simulink model "UnicycleWithSensor"  (R2025b)
settings: Solver=VariableStepAuto  StartTime=0.0  StopTime=200  RelTol=1e-3
values from neighbouring files (symbols this model uses):
  l = 0.5    [go2goalWithSensor.m]
  P = 10    [go2goalWithSensor.m]
  r = 0.1    [go2goalWithSensor.m]
  thetainit = 0    [go2goalWithSensor.m]
  tol = 0.1    [go2goalWithSensor.m]
  v = 0.5    [go2goalWithSensor.m]
  xg = gPos(2)    [go2goalWithSensor.m]
  xinit = sPos(2)    [go2goalWithSensor.m]
  yg = gPos(1)    [go2goalWithSensor.m]
  yinit = sPos(1)    [go2goalWithSensor.m]
  Z = ones(SizeX, SizeY)*255    [CreateMaze.m]
libraries: slpidlib x1, simulink_extras x1
settings Model: PacingRate=4  Creator=npn01  LastModifiedBy=kimsv
settings SolverCC: AlgebraicLoopSolver=TrustRegion
settings DebuggingCC: UnconnectedInputMsg=warning  UnconnectedOutputMsg=warning  UnconnectedLineMsg=warning  ArithmeticOperatorsInVariantConditions=warning
settings ModelReferenceCC: EnableRefExpFcnMdlSchedulingChecks=on
settings SFSimCC: CustomCodeUndefinedFunction=UseInterfaceOnly
settings RTWCC: GPUComputeCapability=3.5

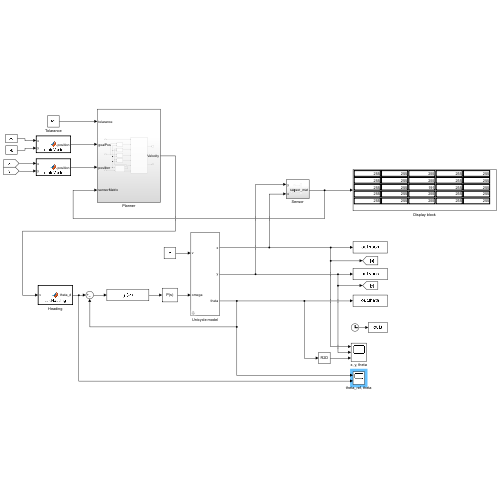
[thumbnail: Simulink's stored preview of the top-level diagram]
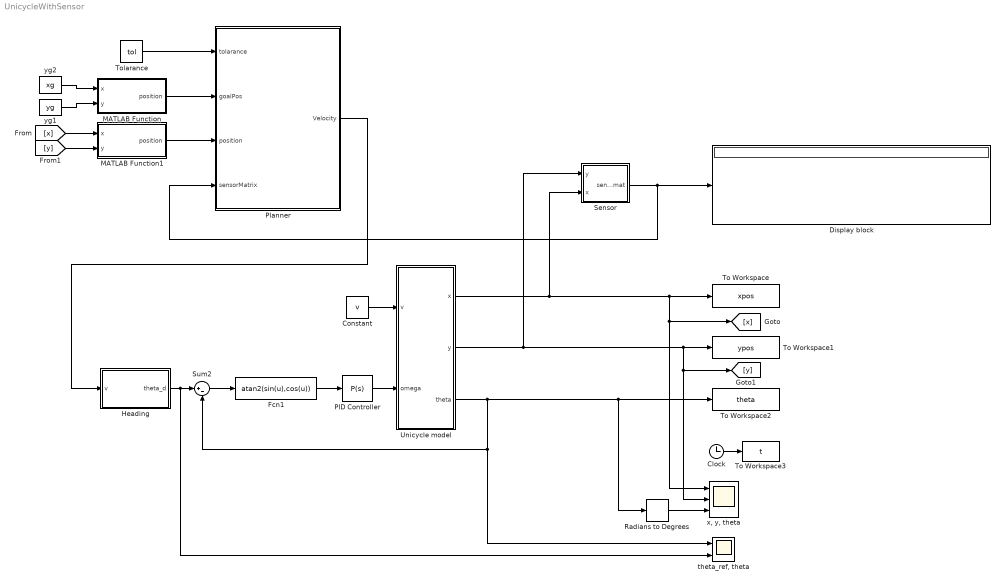
== system UnicycleWithSensor ==
  Clock : Clock
  Constant : Constant  Value=v
  Display block : Display
  Fcn1 : Fcn  Expr=atan2(sin(u),cos(u))
  Heading : MATLAB Function  TreatAsAtomicUnit=on
  MATLAB Function : MATLAB Function  TreatAsAtomicUnit=on
  MATLAB Function1 : MATLAB Function  TreatAsAtomicUnit=on
  PID Controller : slpidlib/PID Controller  Controller=P  Form=Parallel  TimeDomain=Continuous-time  UseExternalTs=off  SampleTime=-1  IntegratorMethod=Forward Euler  FilterMethod=Forward Euler  ControllerParametersSource=internal  P=P  I=0  UseKiTs=off  D=0  UseExternalDerivativeSource=off  N=100  UseFilter=on  TunerSelectOption=Transfer Function Based (PID Tuner App)  InitialConditionSource=internal  InitialConditionForIntegrator=0  InitialConditionForFilter=0  DifferentiatorICPrevScaledInput=0  ExternalReset=none  TrackingMode=off  Kt=1  LimitOutput=off  SatLimitsSource=internal  UpperSaturationLimit=inf  LowerSaturationLimit=-inf  LinearizeAsGain=on  AntiWindupMode=none  Kb=1  LimitIntegrator=off  UpperIntegratorSaturationLimit=inf  LowerIntegratorSaturationLimit=-inf  POutMin=[]  POutMax=[]  IOutMin=[]  IOutMax=[]  DOutMin=[]  DOutMax=[]  NOutMin=[]  NOutMax=[]  SumOutMin=[]  SumOutMax=[]  SaturationOutMin=[]  SaturationOutMax=[]  PParamMin=[]  PParamMax=[]  IParamMin=[]  IParamMax=[]  DParamMin=[]  DParamMax=[]  NParamMin=[]  NParamMax=[]  KbParamMin=[]  KbParamMax=[]  KtParamMin=[]  KtParamMax=[]  KbOutMin=[]  KbOutMax=[]  KtOutMin=[]  KtOutMax=[]  IntegratorOutMin=[]  IntegratorOutMax=[]  FilterOutMin=[]  FilterOutMax=[]  SumI1OutMin=[]  SumI1OutMax=[]  SumI2OutMin=[]  SumI2OutMax=[]  SumI3OutMin=[]  SumI3OutMax=[]  SumI4OutMin=[]  SumI4OutMax=[]  SumDOutMin=[]  SumDOutMax=[]  DifferentiatorOutMin=[]  DifferentiatorOutMax=[]  FilterDiffOutCoefMin=[]  FilterDiffOutCoefMax=[]  ReciprocalOutMin=[]  ReciprocalOutMax=[]  SumDenOutMin=[]  SumDenOutMax=[]  SumNumOutMin=[]  SumNumOutMax=[]  DivideOutMin=[]  DivideOutMax=[]  UdiffTsProdOutMin=[]  UdiffTsProdOutMax=[]  NTsProdOutMin=[]  NTsProdOutMax=[]  UintegralTsProdOutMin=[]  UintegralTsProdOutMax=[]  UngainTsProdOutMin=[]  UngainTsProdOutMax=[]  ClampingZeroOutDataTypeStr=Inherit: Inherit via back propagation  ClampingZeroOutMin=[]  ClampingZeroOutMax=[]  FilterDenConstantOutDataTypeStr=Inherit: Inherit via back propagation  FilterDenConstantOutMin=[]  FilterDenConstantOutMax=[]  PCopyOutDataTypeStr=Inherit: Inherit via back propagation  PCopyOutMin=[]  PCopyOutMax=[]  NCopyOutDataTypeStr=Inherit: Inherit via back propagation  NCopyOutMin=[]  NCopyOutMax=[]  IntegratorContinuousStateAttributes=''  IntegratorStateMustResolveToSignalObject=off  IntegratorRTWStateStorageClass=Auto  FilterContinuousStateAttributes=''  FilterStateMustResolveToSignalObject=off  FilterRTWStateStorageClass=Auto  ParallelPVariant=InternalParameters  IdealPVariant=Disabled  IVariant=Disabled  DVariant=Disabled  IntegratorVariant=Disabled  SatVariant=Disabled  AWVariant=Disabled  PCopyVariant=Disabled  TRVariant=Disabled  FdbkBlocksVariant=Forward  IdealPFdbkVariant=Disabled  SatFdbkVariant=Disabled  DerivativeFilterVariant=Disabled  NVariant=Disabled  NCopyVariant=Disabled_SignalSpec  FilterICVariant=Disabled  IntegratorICVariant=Disabled  ExternalResetVariant=Disabled  TRSumVariant=Passthrough  SumFdbkVariant=Disabled  SumVariant=Passthrough_P  TsampFilterVariant=InternalTs  TsampNgainVariant=Passthrough  TsampIntegralVariant=Disabled_SignalSpec  ExternalSaturationOutDataTypeStr=Inherit: Same as second input  DerivativeSourceVariant=Disabled  PreIntVariant=InternalPreInt
  Planner : Subsystem
  Radians to Degrees : simulink_extras/Transformations/Radians to Degrees
  Sensor : Subsystem
  Sum2 : Sum  Inputs=|+-
  To Workspace : ToWorkspace  VariableName=xpos  SampleTime=-1
  To Workspace1 : ToWorkspace  VariableName=ypos  SampleTime=-1
  To Workspace2 : ToWorkspace  VariableName=theta  SampleTime=-1
  To Workspace3 : ToWorkspace  VariableName=t  SampleTime=-1
      settings: Save2DSignal=2-D array (concatenate along first dimension)
  Tolarance : Constant  Value=tol
  Unicycle model : Subsystem  mask{x0=xinit, y0=yinit, theta0=thetainit}
      mask DialogControl Control4 Prompt: Enter x initial position
      mask DialogControl Control2 Prompt: Enter y initial position
      mask DialogControl Control3 Prompt: Enter initial theta angle
      mask DialogControl Control6 Prompt: Any text you want
  "theta_ref, theta" : Scope  NumInputPorts=2
      settings: ActiveDisplayYMinimum=-3.6016873206532476  ActiveDisplayYMaximum=5.63573543998936
  "x, y, theta" : Scope  NumInputPorts=3
      settings: ActiveDisplayString=3  ActiveDisplayYMinimum=-134.97289881582088  ActiveDisplayYMaximum=314.97179029887303  YLabel=Angle (Degrees)  DataLoggingVariableName=ScopeData2
  yg1 : Constant  Value=yg
  yg2 : Constant  Value=xg
  wires:
  Unicycle model/1(x) -> Sensor/2(x), [x], "x, y, theta"/1, To Workspace/1
  Unicycle model/2(y) -> [y], "x, y, theta"/2, To Workspace1/1, Sensor/1(y)
  Unicycle model/3(theta) -> Radians to Degrees/1, To Workspace2/1, Sum2/2, "theta_ref, theta"/1
  PID Controller/1 -> Unicycle model/2(omega)
  Clock/1 -> To Workspace3/1
  Sensor/1(sensor_mat) -> Planner/4(sensorMatrix), Display block/1
  yg1/1 -> MATLAB Function/2(y)
  MATLAB Function/1(position) -> Planner/2(goalPos)
  MATLAB Function1/1(position) -> Planner/3(position)
  Planner/1(Velocity) -> Heading/1(v)
  Heading/1(theta_d) -> "theta_ref, theta"/2, Sum2/1
  [x] -> MATLAB Function1/1(x)
  [y] -> MATLAB Function1/2(y)
  Sum2/1 -> Fcn1/1
  Fcn1/1 -> PID Controller/1
  yg2/1 -> MATLAB Function/1(x)
  Radians to Degrees/1 -> "x, y, theta"/3
  Constant/1 -> Unicycle model/1(v)
  Tolarance/1 -> Planner/1(tolarance)

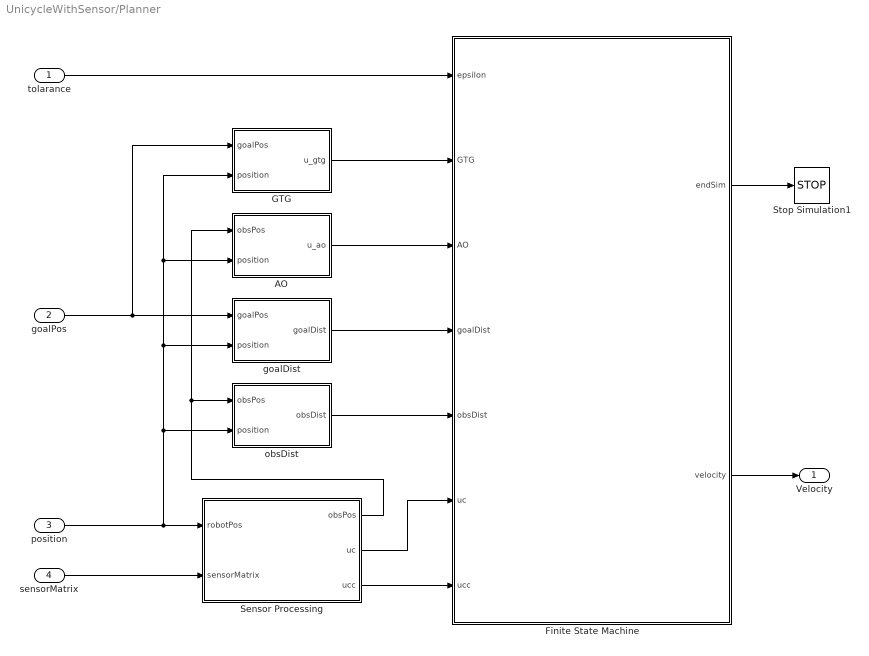
== system UnicycleWithSensor/Planner ==
  tolarance : Inport
  goalPos : Inport  Port=2
  position : Inport  Port=3
  sensorMatrix : Inport  Port=4
  AO : MATLAB Function  TreatAsAtomicUnit=on
  Finite State Machine : Stateflow chart  TreatAsAtomicUnit=on
      settings: PortSchema="{\"entries\":[{\"content\":{\"sides\":[{\"content\":{\"connectorIds\":[\"In7\",\"In3\",\"In4\",\"In5\",\"In6\",\"In1\",\"In2\"]},\"type\":\"ConnectorPlacement.EquallySpacedRectSide\",\"uuid\":\"7bddc3d5-5a53-4f00-97fb-67b91d40fd27\"},{\"content\":{\"connectorIds\":[\"Out2\",\"Out1\"],\"side\":\"RIGHT\"},\"type\":\"ConnectorPlacement.EquallySpacedRectSide\",\"uuid\":\"08b6080d-a441-42a3-994a-8d28211d42e3\"},{\"content\":{\"side\":\"TOP\"},\"type\":\"ConnectorPlacement.EquallySpacedRectSide\",\"uuid\":\"62170fc2-3338-4bec-a116-8b710f92c3e1\"}]},\"type\":\"ConnectorPlacement.EquallySpacedConnector\",\"uuid\":\"879b9b83-d19d-42da-995b-71e8b8a5ae61\"}],\"packageUris\":[\"http://schema.mathworks.com/mf0/Connector/R2020b\"],\"version\":\"1.0\"}"
  GTG : MATLAB Function  TreatAsAtomicUnit=on
  Sensor Processing : MATLAB Function  TreatAsAtomicUnit=on
  Stop Simulation1 : Stop
  goalDist : MATLAB Function  TreatAsAtomicUnit=on
  obsDist : MATLAB Function  TreatAsAtomicUnit=on
  Velocity : Outport
  wires:
  position/1 -> Sensor Processing/1(robotPos), obsDist/2(position), goalDist/2(position), AO/2(position), GTG/2(position)
  goalPos/1 -> GTG/1(goalPos), goalDist/1(goalPos)
  Sensor Processing/2(uc) -> Finite State Machine/1(uc)
  Sensor Processing/3(ucc) -> Finite State Machine/2(ucc)
  sensorMatrix/1 -> Sensor Processing/2(sensorMatrix)
  Sensor Processing/1(obsPos) -> AO/1(obsPos), obsDist/1(obsPos)
  GTG/1(u_gtg) -> Finite State Machine/3(GTG)
  goalDist/1(goalDist) -> Finite State Machine/5(goalDist)
  obsDist/1(obsDist) -> Finite State Machine/6(obsDist)
  Finite State Machine/2(endSim) -> Stop Simulation1/1
  Finite State Machine/1(velocity) -> Velocity/1
  tolarance/1 -> Finite State Machine/7(epsilon)
  AO/1(u_ao) -> Finite State Machine/4(AO)

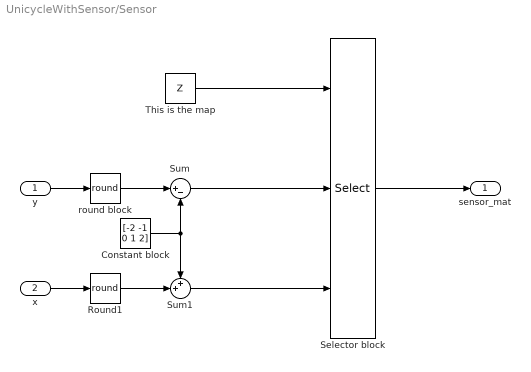
== system UnicycleWithSensor/Sensor ==
  y : Inport
  x : Inport  Port=2
  Constant block : Constant  Value=[-2 -1 0 1 2]
  Round1 : Rounding  Operator=round
  Selector block : Selector  NumberOfDimensions=2  InputPortWidth=3  IndexOptions=Index vector (port),Index vector (port)  Indices=[1 3],1  OutputSizes=1,1
  Sum : Sum  Inputs=|+-  OutDataTypeStr=int32  RndMeth=Round
  Sum1 : Sum  Inputs=++|  OutDataTypeStr=int32  RndMeth=Round
  This is the map : Constant  Value=Z  VectorParams1D=off
  round block : Rounding  Operator=round
  sensor_mat : Outport
  wires:
  This is the map/1 -> Selector block/1
  Constant block/1 -> Sum1/1, Sum/2
  Sum/1 -> Selector block/2
  Sum1/1 -> Selector block/3
  Selector block/1 -> sensor_mat/1
  y/1 -> round block/1
  round block/1 -> Sum/1
  x/1 -> Round1/1
  Round1/1 -> Sum1/2

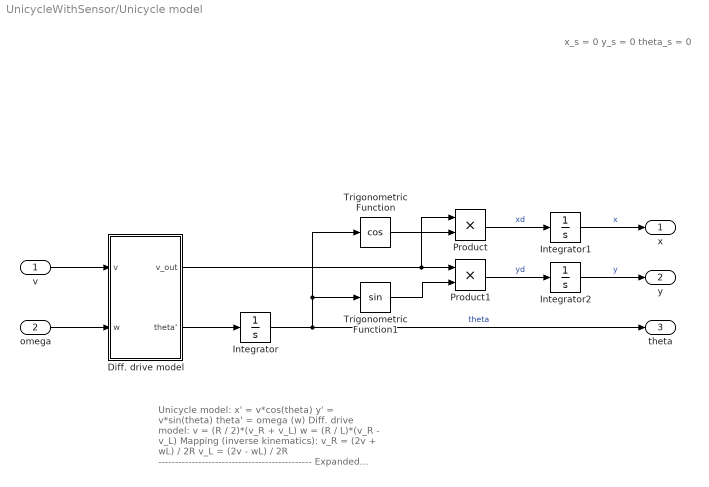
== system UnicycleWithSensor/Unicycle model ==
  note: x_s = 0
      | y_s = 0
      | theta_s = 0
  note: Unicycle model:
      | x' = v*cos(theta)
      | y' = v*sin(theta)
      | theta' = omega (w)
      |
      | Diff. drive model:
      | v = (R / 2)*(v_R + v_L)
      | w = (R / L)*(v_R - v_L)
      |
      | Mapping (inverse kinematics):
      | v_R = (2v + wL) / 2R
      | v_L = (2v - wL) / 2R
      | ----------------------------------------------
      | Expanded unicycle model:
      | x' =  ((R / 2)*(v_R + v_L))*cos(theta)
      | y' =  ((R / 2)*(v_R + v_L))*sin(theta)
      | theta' =  (R / L)*(v_R - v_L)
  v : Inport
  omega : Inport  Port=2
  Diff. drive model : Subsystem
  Integrator : Integrator  InitialCondition=theta0
  Integrator1 : Integrator  InitialCondition=x0
  Integrator2 : Integrator  InitialCondition=y0
  Product : Product
  Product1 : Product
  Trigonometric Function : Trigonometry  Operator=cos
  Trigonometric Function1 : Trigonometry
  x : Outport
  y : Outport  Port=2
  theta : Outport  Port=3
  wires:
  Product1/1 -> Integrator2/1  "yd"
  Integrator2/1 -> y/1  "y"
  v/1 -> Diff. drive model/1(v)
  Integrator/1 -> Trigonometric Function/1, Trigonometric Function1/1, theta/1  "theta"
  Product/1 -> Integrator1/1  "xd"
  omega/1 -> Diff. drive model/2(w)
  Trigonometric Function/1 -> Product/2
  Integrator1/1 -> x/1  "x"
  Trigonometric Function1/1 -> Product1/2
  Diff. drive model/1(v_out) -> Product/1, Product1/1
  Diff. drive model/2(theta') -> Integrator/1

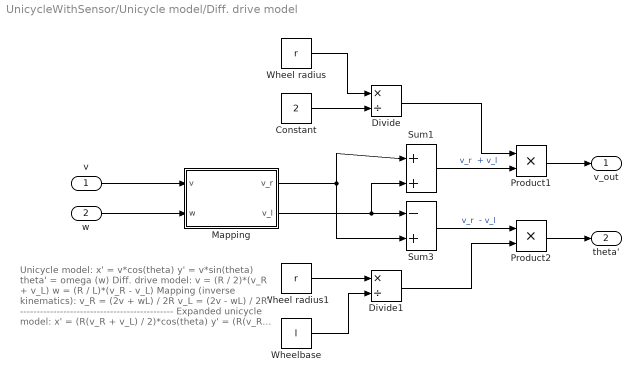
== system UnicycleWithSensor/Unicycle model/Diff. drive model ==
  note: Unicycle model:
      | x' = v*cos(theta)
      | y' = v*sin(theta)
      | theta' = omega (w)
      |
      | Diff. drive model:
      | v = (R / 2)*(v_R + v_L)
      | w = (R / L)*(v_R - v_L)
      |
      | Mapping (inverse kinematics):
      | v_R = (2v + wL) / 2R
      | v_L = (2v - wL) / 2R
      | ----------------------------------------------
      | Expanded unicycle model:
      | x' =  (R(v_R + v_L) / 2)*cos(theta)
      | y' =  (R(v_R + v_L) / 2)*sin(theta)
      | theta' =  R(v_R - v_L) / L
  v : Inport
  w : Inport  Port=2
  Constant : Constant  Value=2
  Divide : Product  Inputs=*/
  Divide1 : Product  Inputs=*/
  Mapping : Subsystem
  Product1 : Product
  Product2 : Product
  Sum1 : Sum  Inputs=+|+
  Sum3 : Sum  Inputs=-+
  Wheel radius : Constant  Value=r
  Wheel radius1 : Constant  Value=r
  Wheelbase : Constant  Value=l
  v_out : Outport
  theta' : Outport  Port=2
  wires:
  v/1 -> Mapping/1(v)
  w/1 -> Mapping/2(w)
  Wheel radius/1 -> Divide/1
  Constant/1 -> Divide/2
  Mapping/1(v_r) -> Sum3/2, Sum1/1
  Mapping/2(v_l) -> Sum1/2, Sum3/1
  Wheel radius1/1 -> Divide1/1
  Wheelbase/1 -> Divide1/2
  Divide1/1 -> Product2/2
  Product2/1 -> theta'/1
  Sum1/1 -> Product1/2  "v_r  + v_l"
  Divide/1 -> Product1/1
  Product1/1 -> v_out/1
  Sum3/1 -> Product2/1  "v_r  - v_l"

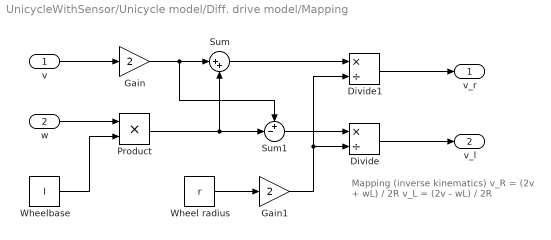
== system UnicycleWithSensor/Unicycle model/Diff. drive model/Mapping ==
  note: Mapping (inverse kinematics)
      | v_R = (2v + wL) / 2R
      | v_L = (2v - wL) / 2R
  v : Inport
  w : Inport  Port=2
  Divide : Product  Inputs=*/
  Divide1 : Product  Inputs=*/
  Gain : Gain  Gain=2
  Gain1 : Gain  Gain=2
  Product : Product
  Sum : Sum  Inputs=|++
  Sum1 : Sum  Inputs=+-|
  Wheel radius : Constant  Value=r
  Wheelbase : Constant  Value=l
  v_r : Outport
  v_l : Outport  Port=2
  wires:
  v/1 -> Gain/1
  Product/1 -> Sum1/2, Sum/2
  w/1 -> Product/1
  Wheelbase/1 -> Product/2
  Wheel radius/1 -> Gain1/1
  Sum/1 -> Divide1/1
  Sum1/1 -> Divide/1
  Gain1/1 -> Divide/2, Divide1/2
  Divide1/1 -> v_r/1
  Divide/1 -> v_l/1
  Gain/1 -> Sum1/1, Sum/1

== matlab function UnicycleWithSensor/Planner/GTG ==
  data: goalPos input; u_gtg output; position input
function u_gtg = fcn(goalPos, position)
u_gtg = (goalPos - position) / (norm(goalPos - position) + eps);

end

== matlab function UnicycleWithSensor/Planner/AO ==
  data: obsPos input; u_ao output; position input
function u_ao = fcn(obsPos, position)
u_ao = (position - obsPos) / (norm(position - obsPos) + eps);

end

== stateflow chart UnicycleWithSensor/Planner/Finite State Machine ==
  state stop_state
    entry:
    endSim = true;
  state u_gtg_state
    entry:
    velocity = GTG;
    during:
    velocity = GTG;
    dot_gtg_ucc = dot(GTG, ucc);
    dot_gtg_uc = dot(GTG, uc);
  state uc_fw_state
    entry:
    d = goalDist;
    velocity = uc;
    during:
    velocity = uc;
    dot_uao_gtg = dot(AO, GTG);
  state ucc_fw_state
    entry:
    d = goalDist;
    velocity = ucc;
    during:
    velocity = ucc;
    dot_uao_gtg = dot(AO, GTG);
  state u_ao_state
    entry:
    velocity = AO;
    during:
    velocity = AO;
    dot_gtg_uc = dot(GTG, uc);
    dot_gtg_ucc = dot(GTG, ucc);
  u_gtg_state -> stop_state [order 3] : [goalDist <= epsilon]
  u_gtg_state -> uc_fw_state [order 2] : [obsDist < delta1 && dot_gtg_uc > 0]
  (default) -> u_gtg_state
  uc_fw_state -> u_gtg_state [order 1] : [goalDist < d && dot_uao_gtg > 0]
  ucc_fw_state -> u_gtg_state [order 1] : [goalDist < d && dot_uao_gtg > 0]
  u_gtg_state -> ucc_fw_state [order 1] : [obsDist < delta1 && dot_gtg_ucc > 0]
  uc_fw_state -> u_ao_state [order 2] : [obsDist < delta2]
  u_ao_state -> uc_fw_state [order 1] : [obsDist >= delta2 && dot_gtg_uc > 0]
  u_ao_state -> ucc_fw_state [order 2] : [obsDist >= delta2 && dot_gtg_ucc > 0]
  ucc_fw_state -> u_ao_state [order 2] : [obsDist < delta2]
  data: delta1 local =2; delta2 local =0.75; uc input size=[2 1]; ucc input size=[2 1]; dot_gtg_uc local =0; dot_gtg_ucc local =0; velocity output size=[2 1]; d local; dot_uao_gtg local =0; endSim output; GTG input size=[2 1]; AO input size=[2 1]; goalDist input; obsDist input; epsilon input double =0.1

== matlab function UnicycleWithSensor/Planner/goalDist ==
  data: goalPos input; goalDist output; position input
function goalDist = fcn(goalPos, position)
goalDist = norm(position - goalPos);

end

== matlab function UnicycleWithSensor/Planner/obsDist ==
  data: obsPos input; obsDist output; position input
function obsDist = fcn(obsPos, position)
obsDist = norm(position - obsPos);

end

== matlab function UnicycleWithSensor/MATLAB Function1 ==
  data: x input; position output; y input
function position = createVector(x, y)

position = [x; y];

end

== matlab function UnicycleWithSensor/MATLAB Function ==
  data: x input; position output; y input
function position = createVector(x, y)

position = [x; y];

end

== matlab function UnicycleWithSensor/Planner/Sensor Processing ==
  data: robotPos input; obsPos output; uc output; ucc output; sensorMatrix input
function [obsPos, uc, ucc]  = fcn(robotPos, sensorMatrix)

% Find the obstacle in the 5x5 grid
[r, c] = find(sensorMatrix == 0);

if isempty(r)
        % No obstacle detected
        uc = [0; 0];
        ucc = [0; 0];
        obsPos = [99; 99];
    else
        % Calculate all obstacle (wall) points 
        dist_sq = (c - 3).^2 + (r - 3).^2;

        % Take the nearest obstacle point
        [~, idx] = min(dist_sq);

        % Vector to obstacle in coordinates
        dx = c(idx) - 3;        
        dy = 3 - r(idx);        
        obs_global = [dx; dy]; 
        
        % Global obstacle position
        obsPos = robotPos + obs_global;
        
        % Calculate avoidance vector
        u_AO = -obs_global / (norm(obs_global) + eps);
        
        % Apply the wall gollowing rotations
        uc  = [0, 1; -1, 0] * u_AO;
        ucc = [0, -1; 1, 0] * u_AO;
    end
end

== matlab function UnicycleWithSensor/Heading ==
  data: v input; theta_d output
function theta_d = calcHeading(v)
theta_d = atan2(v(2), v(1));
